simulink model "breathing_rate_adc1"  (R2020b)
settings: Solver=ode15s  StartTime=0.0  StopTime=60  RelTol=1e-3  AbsTol=1e-3  EnableMultiTasking=on
undefined symbols (not defined in the file): sigbuilder_block
libraries: fl_lib x22, nesl_utility x6, ee_lib x4, simulink x1
CloseFcn:
  | try,close(h1_elec_strain_gauge),end
  | clear h1_elec_strain_gauge
  | 
  | clear logsout_elec_strain_gauge
  | clear simlog_elec_strain_gauge
  | clear tout
Description:
  | Strain Gauge and Wheatstone Bridge
  | 
  | Copyright 2008-2018 The MathWorks, Inc.
settings Model: ExtModeAutoUpdateStatusClock=off  Creator=MathWorks  LastModifiedBy=bolic
settings SolverCC: AutoScaleAbsTol=off
settings DataIOCC: MaxDataPoints=10000  ReturnWorkspaceOutputs=off  SignalLoggingName=logsout_elec_strain_gauge  Refine=5
settings OptimizationCC: ExpressionDepthLimit=2147483647  InitFltsAndDblsToZero=on  LifeSpan=inf
settings DebuggingCC: SaveWithParameterizedLinksMsg=none  UnderspecifiedInitializationDetection=Classic  MergeDetectMultiDrivingBlocksExec=none  SignalResolutionControl=TryResolveAllWithWarning  FcnCallInpInsideContextMsg=warning  StateNameClashWarn=warning  SFUnexpectedBacktrackingDiag=warning  SFNoUnconditionalDefaultTransitionDiag=warning  SFExecutionAtInitializationDiag=none  ArithmeticOperatorsInVariantConditions=warning
settings HardwareCC: ProdBitPerPointer=32  ProdBitPerSizeT=32  ProdBitPerPtrDiffT=32  ProdLargestAtomicFloat=None  ProdIntDivRoundTo=Undefined  ProdEndianess=Unspecified  ProdWordSize=32  ProdHWDeviceType=32-bit Generic
settings ModelReferenceCC: PropagateSignalLabelsOutOfModel=off
settings SFSimCC: SimUseLocalCustomCode=off  CustomCodeUndefinedFunction=UseInterfaceOnly
settings RTWCC: RTWUseLocalCustomCode=off
settings CodeAppCC: StateflowObjectComments=on
settings GRTTargetCC: TargetFcnLib=ansi_tfl_tmw.mat  TargetLangStandard=C89/C90 (ANSI)  CombineOutputUpdateFcns=off  GRTInterface=on
settings ConfigComp: CovMetricSettings=dw  CovSaveCumulativeToWorkspaceVar=on  CovSaveSingleToWorkspaceVar=on  CovExternalEMLEnable=off  CovSFcnEnable=off
settings SimscapeCC: SimscapeLogType=all  SimscapeLogSimulationStatistics=on  SimscapeLogName=simlog_elec_strain_gauge  SimscapeLogDataHistory=10000

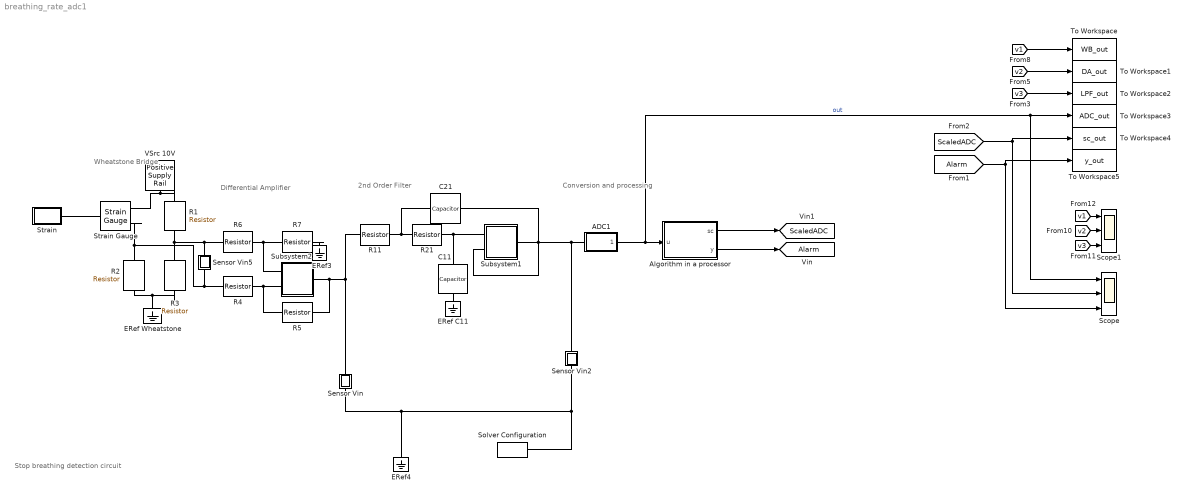
== system breathing_rate_adc1 ==
  note: Differential Amplifier
  note: Wheatstone
      | Bridge
  note: Stop breathing detection circuit
  note: 2nd Order Filter
  note: Conversion and processing
  ADC1 : Subsystem  mask(ADC){fs=80, N=12, vmax=5, ileak=1e-9, C=10e-12}
      mask prompts: fs "Sampling rate (Hz)"; N "Number of bits"; vmax "Input voltage for max output (V)"; ileak "Leakage current (A)"; C "Pin capacitance (F)"
      mask help: Simplified analog-to-digital converter
  Algorithm in a processor : MATLAB Function  TreatAsAtomicUnit=on
  C11 : fl_lib/Electrical/Electrical Elements/Capacitor  c=800 nF  r=0 Ohm  g=0 1/Ohm  i_specify=off  i_priority=High  i=0 A  i_nominal_specify=off  i_nominal_unit=A  i_nominal_value=1  v_specify=off  v_priority=High  v=0 V  v_nominal_specify=off  v_nominal_unit=V  v_nominal_value=1  vc_specify=off  vc_priority=High  vc=0 V  vc_nominal_specify=off  vc_nominal_unit=V  vc_nominal_value=1
      settings: SourceProductName=Foundation Library
  C21 : fl_lib/Electrical/Electrical Elements/Capacitor  c=800 nF  r=0 Ohm  g=0 1/Ohm  i_specify=off  i_priority=High  i=0 A  i_nominal_specify=off  i_nominal_unit=A  i_nominal_value=1  v_specify=off  v_priority=High  v=0 V  v_nominal_specify=off  v_nominal_unit=V  v_nominal_value=1  vc_specify=off  vc_priority=High  vc=0 V  vc_nominal_specify=off  vc_nominal_unit=V  vc_nominal_value=1
      settings: SourceProductName=Foundation Library
  ERef C11 : fl_lib/Electrical/Electrical Elements/Electrical Reference
      settings: SourceProductName=Foundation Library
  ERef Wheatstone : fl_lib/Electrical/Electrical Elements/Electrical Reference
      settings: SourceProductName=Foundation Library
  ERef3 : fl_lib/Electrical/Electrical Elements/Electrical Reference
      settings: SourceProductName=Foundation Library
  ERef4 : fl_lib/Electrical/Electrical Elements/Electrical Reference
      settings: SourceProductName=Foundation Library
  R{1..4,6} (5 alike) : fl_lib/Electrical/Electrical Elements/Resistor  R=100 Ohm  i_specify=off  i_priority=High  i=0 A  i_nominal_specify=off  i_nominal_unit=A  i_nominal_value=1  v_specify=off  v_priority=High  v=0 V  v_nominal_specify=off  v_nominal_unit=V  v_nominal_value=1
      settings: SourceProductName=Foundation Library
  R11 : fl_lib/Electrical/Electrical Elements/Resistor  R=10 kOhm  i_specify=off  i_priority=High  i=0 A  i_nominal_specify=off  i_nominal_unit=A  i_nominal_value=1  v_specify=off  v_priority=High  v=0 V  v_nominal_specify=off  v_nominal_unit=V  v_nominal_value=1
      settings: SourceProductName=Foundation Library
  R21 : fl_lib/Electrical/Electrical Elements/Resistor  R="10  kOhm"  i_specify=off  i_priority=High  i=0 A  i_nominal_specify=off  i_nominal_unit=A  i_nominal_value=1  v_specify=off  v_priority=High  v=0 V  v_nominal_specify=off  v_nominal_unit=V  v_nominal_value=1
      settings: SourceProductName=Foundation Library
  R5 : fl_lib/Electrical/Electrical Elements/Resistor  R=10 kOhm  i_specify=off  i_priority=High  i=0 A  i_nominal_specify=off  i_nominal_unit=A  i_nominal_value=1  v_specify=off  v_priority=High  v=0 V  v_nominal_specify=off  v_nominal_unit=V  v_nominal_value=1
      settings: SourceProductName=Foundation Library
  R7 : fl_lib/Electrical/Electrical Elements/Resistor  R=10 kOhm  i_specify=off  i_priority=High  i=0 A  i_nominal_specify=off  i_nominal_unit=A  i_nominal_value=1  v_specify=off  v_priority=High  v=0 V  v_nominal_specify=off  v_nominal_unit=V  v_nominal_value=1
      settings: SourceProductName=Foundation Library
  Scope : Scope  NumInputPorts=3
  Scope1 : Scope  NumInputPorts=3
  Sensor Vin : Subsystem
      mask Display: disp('v')
  Sensor Vin2 : Subsystem
      mask Display: disp('v')
  Sensor Vin5 : Subsystem
      mask Display: disp('v')
  Solver Configuration : nesl_utility/Solver Configuration  PhysicalDomain=network_engine_domain  SubClassName=solver  LeftPortType=input  RightPortType=generic  Tones=[]  Harmonics=[]  SimulateNoise=off  Profile=off  UseLocalSampling=off  EnableSwitchedLinearOptims=on  FrequencyDomain=off  UseCCode=off  RelTol=0.001  AbsTol=1e-06  MinStep=1e-09  ToWorkspace=off  RevertToSquareIcSolve=off  NumHomotopyIterations=100  PhasorMode=off  PhasorModeNumHarmonics=1  DoDC=off  ResidualTolerance=1e-9  UseLocalSolver=off  LocalSolverChoice=NE_BACKWARD_EULER_ADVANCER  LocalSolverSampleTime=.001  DoFixedCost=off  MaxNonlinIter=3  MaxModeIter=2  ComputeImpulses=off  ImpulseIterations=2  LinearAlgebra=auto  EquationFormulation=NE_TIME_EF  DelaysMemoryBudget=1024  AutomaticFiltering=on  FilteringTimeConstant=0.001  PartitionStorageMethod=AS_NEEDED  PartitionMemoryBudget=1024  PartitionMethod=FAST
  Strain : Subsystem
      mask Display: disp('Input')
  Strain Gauge : ee_lib/Sensors & Transducers/Strain Gauge  R=100 Ohm  K=2
      settings: SourceProductBaseCode=PS  InternalSimscapePortConfiguration="{\"Bottom\":[],\"Left\":[{\"id\":\"E\",\"label\":\"E\",\"type\":\"input\"}],\"Right\":[{\"id\":\"p\",\"label\":\"+\",\"type\":\"foundation.electrical.electrical\"},{\"id\":\"n\",\"label\":\"-\",\"type\":\"foundation.electrical.electrical\"}],\"Top\":[]}"
  Subsystem1 : Subsystem
      mask Display: image('op_amp_plus_up.png')
  Subsystem2 : Subsystem
      mask Display: image('op_amp_plus_up.png')
  To Workspace : ToWorkspace  VariableName=WB_out  SaveFormat=Timeseries  SampleTime=-1
  To Workspace1 : ToWorkspace  VariableName=DA_out  SaveFormat=Timeseries  SampleTime=-1
  To Workspace2 : ToWorkspace  VariableName=LPF_out  SaveFormat=Timeseries  SampleTime=-1
  To Workspace3 : ToWorkspace  VariableName=ADC_out  SaveFormat=Timeseries  SampleTime=-1
  To Workspace4 : ToWorkspace  VariableName=sc_out  SaveFormat=Timeseries  SampleTime=-1
  To Workspace5 : ToWorkspace  VariableName=y_out  SaveFormat=Timeseries  SampleTime=-1
  VSrc 10V : ee_lib/Sources/Positive Supply Rail  v0=5 V
      settings: SourceProductBaseCode=PS  InternalSimscapePortConfiguration="{\"Bottom\":[],\"Left\":[],\"Right\":[{\"id\":\"p\",\"label\":\"\",\"type\":\"foundation.electrical.electrical\"}],\"Top\":[]}"
  tag scope: Alarm=global, ScaledADC=global
  wires:
  [v1] -> To Workspace/1
  [v2] -> To Workspace1/1
  [v3] -> To Workspace2/1
  [v2] -> Scope1/2
  [v3] -> Scope1/3
  [v1] -> Scope1/1
  ADC1/1(Out_Int) -> Scope/1, To Workspace3/1, Algorithm in a processor/1(u)  "out"
  Algorithm in a processor/2(y) -> [Alarm]
  Algorithm in a processor/1(sc) -> [ScaledADC]
  [Alarm] -> To Workspace5/1, Scope/3
  [ScaledADC] -> To Workspace4/1, Scope/2
  connections:
  R1/LConn1 -- Strain Gauge/RConn1 -- VSrc 10V/RConn1
  Strain Gauge/RConn2 -- Sensor Vin5/LConn1 -- R4/LConn1 -- R2/LConn1
  R1/RConn1 -- R6/LConn1 -- Sensor Vin5/RConn1 -- R3/LConn1
  R3/RConn1 -- R2/RConn1 -- ERef Wheatstone/LConn1
  R4/RConn1 -- Subsystem2/LConn2 -- R5/LConn1
  R5/RConn1 -- R11/LConn1 -- Sensor Vin/RConn1 -- Subsystem2/RConn1
  R6/RConn1 -- Subsystem2/LConn1 -- R7/LConn1
  R7/RConn1 -- ERef3/LConn1
  ERef4/LConn1 -- Solver Configuration/RConn1 -- Sensor Vin2/LConn1 -- Sensor Vin/LConn1
  C11/LConn1 -- Subsystem1/LConn1 -- R21/RConn1
  Sensor Vin2/RConn1 -- ADC1/LConn1 -- Subsystem1/LConn2 -- C21/RConn1 -- Subsystem1/RConn1
  C21/LConn1 -- R21/LConn1 -- R11/RConn1
  ERef C11/LConn1 -- C11/RConn1
  Strain/RConn1 -- Strain Gauge/LConn1

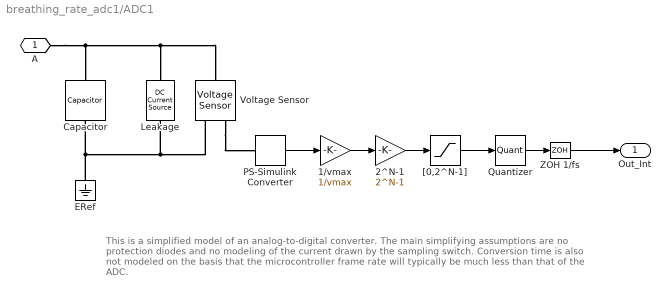
== system breathing_rate_adc1/ADC1 ==
  note: This is a simplified model of an analog-to-digital converter. The main simplifying assumptions
      | are no protection diodes and no modeling of the current drawn by the sampling switch.
      | Conversion time is also not modeled on the basis that the microcontroller frame rate will
      | typically be much less than that of the ADC.
  1/vmax : Gain  Gain=1/vmax
  2^N-1 : Gain  Gain=2^N-1
  Capacitor : fl_lib/Electrical/Electrical Elements/Capacitor  c=1e-6 F  r=1e-6 Ohm  g=0 1/Ohm  i_specify=off  i_priority=High  i=0 A  i_nominal_specify=off  i_nominal_unit=A  i_nominal_value=1  v_specify=off  v_priority=High  v=0 V  v_nominal_specify=off  v_nominal_unit=V  v_nominal_value=1  vc_specify=on  vc_priority=High  vc=0 V  vc_nominal_specify=off  vc_nominal_unit=V  vc_nominal_value=1
      settings: SourceProductName=Foundation Library
  ERef : fl_lib/Electrical/Electrical Elements/Electrical Reference
      settings: SourceProductName=Foundation Library
  Leakage : fl_lib/Electrical/Electrical Sources/DC Current Source  i0=ileak A
      settings: SourceProductName=Foundation Library  InternalSimscapePortConfiguration="{\"Bottom\":[],\"Left\":[{\"id\":\"p\",\"label\":\"\",\"type\":\"foundation.electrical.electrical\"}],\"Right\":[{\"id\":\"n\",\"label\":\"\",\"type\":\"foundation.electrical.electrical\"}],\"Top\":[]}"
  PS-Simulink Converter : nesl_utility/PS-Simulink Converter  PhysicalDomain=network_engine_domain  SubClassName=ps_output  LeftPortType=input  RightPortType=output  PseudoPeriodic=off  Frequencies=[]  Unit=V  AffineConversion=off
  Quantizer : Quantizer  QuantizationInterval=1
  Voltage Sensor : fl_lib/Electrical/Electrical Sensors/Voltage Sensor
      settings: SourceProductName=Foundation Library
  ZOH 1/fs : ZeroOrderHold  SampleTime=1/fs
  "[0,2^N-1]" : Saturate  UpperLimit=2^N-1  LowerLimit=0
  A : PMIOPort  Side=Left
  Out_Int : Outport  VectorParamsAs1DForOutWhenUnconnected=off
  wires:
  "[0,2^N-1]"/1 -> Quantizer/1
  1/vmax/1 -> 2^N-1/1
  2^N-1/1 -> "[0,2^N-1]"/1
  PS-Simulink Converter/1 -> 1/vmax/1
  ZOH 1/fs/1 -> Out_Int/1
  Quantizer/1 -> ZOH 1/fs/1
  connections:
  A/RConn1 -- Voltage Sensor/LConn1 -- Leakage/RConn1 -- Capacitor/LConn1
  ERef/LConn1 -- Voltage Sensor/RConn2 -- Leakage/LConn1 -- Capacitor/RConn1
  Voltage Sensor/RConn1 -- PS-Simulink Converter/LConn1

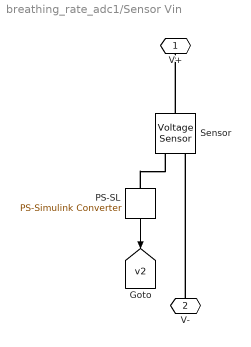
== system breathing_rate_adc1/Sensor Vin ==
  PS-SL : nesl_utility/PS-Simulink Converter  PhysicalDomain=network_engine_domain  SubClassName=ps_output  LeftPortType=input  RightPortType=output  PseudoPeriodic=off  Frequencies=[]  Unit=1  AffineConversion=off
  Sensor : fl_lib/Electrical/Electrical Sensors/Voltage Sensor
      settings: SourceProductName=Foundation Library
  V+ : PMIOPort  Side=Right
  V- : PMIOPort  Port=2  Side=Left
  tag scope: v2=global
  wires:
  PS-SL/1 -> [v2]
  connections:
  PS-SL/LConn1 -- Sensor/RConn1
  Sensor/LConn1 -- V+/RConn1
  V-/RConn1 -- Sensor/RConn2

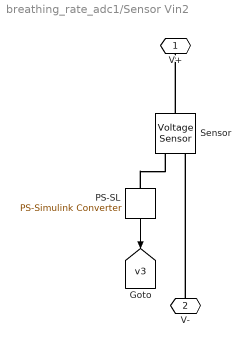
== system breathing_rate_adc1/Sensor Vin2 ==
  PS-SL : nesl_utility/PS-Simulink Converter  PhysicalDomain=network_engine_domain  SubClassName=ps_output  LeftPortType=input  RightPortType=output  PseudoPeriodic=off  Frequencies=[]  Unit=1  AffineConversion=off
  Sensor : fl_lib/Electrical/Electrical Sensors/Voltage Sensor
      settings: SourceProductName=Foundation Library
  V+ : PMIOPort  Side=Right
  V- : PMIOPort  Port=2  Side=Left
  tag scope: v3=global
  wires:
  PS-SL/1 -> [v3]
  connections:
  PS-SL/LConn1 -- Sensor/RConn1
  Sensor/LConn1 -- V+/RConn1
  V-/RConn1 -- Sensor/RConn2

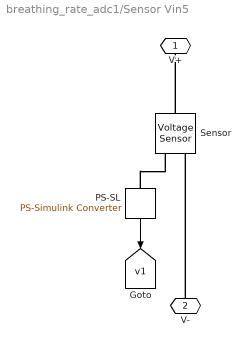
== system breathing_rate_adc1/Sensor Vin5 ==
  PS-SL : nesl_utility/PS-Simulink Converter  PhysicalDomain=network_engine_domain  SubClassName=ps_output  LeftPortType=input  RightPortType=output  PseudoPeriodic=off  Frequencies=[]  Unit=1  AffineConversion=off
  Sensor : fl_lib/Electrical/Electrical Sensors/Voltage Sensor
      settings: SourceProductName=Foundation Library
  V+ : PMIOPort  Side=Right
  V- : PMIOPort  Port=2  Side=Left
  tag scope: v1=global
  wires:
  PS-SL/1 -> [v1]
  connections:
  PS-SL/LConn1 -- Sensor/RConn1
  Sensor/LConn1 -- V+/RConn1
  V-/RConn1 -- Sensor/RConn2

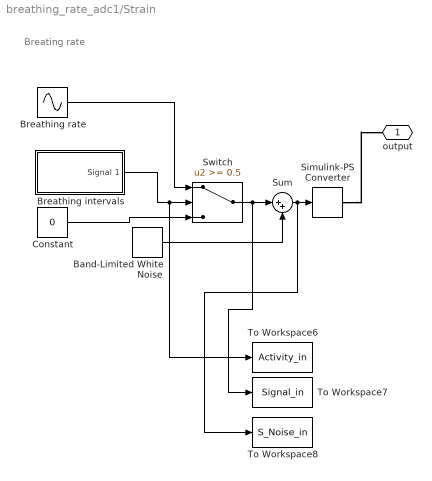
== system breathing_rate_adc1/Strain ==
  note: Breating rate
  Band-Limited White Noise : simulink/Sources/Band-Limited White Noise  Cov=[0.0000000001]  Ts=0.001  seed=[23341]
  Breathing intervals : Subsystem  Tag=STV Subsys  LoadFcn=sigbuilder_block('load');  StartFcn=sigbuilder_block('start');  StopFcn=sigbuilder_block('stop');  ClipboardFcn=sigbuilder_block('clipboard');  mask(Sigbuilder block){tuvar=[0:10]}
      mask help: Simulink:masks:SigbuilderBlock_MD
      mask init:
      | if ~strcmp(get_param(bdroot(gcbh),'SimulationStatus'),'stopped') tuvar = sigbuilder_block('maskInit'); end
      settings: CopyFcn=sigbuilder_block('copy');  DeleteFcn=sigbuilder_block('delete');  ModelCloseFcn=sigbuilder_block('modelClose');  PreSaveFcn=sigbuilder_block('preSave');  PauseFcn=sigbuilder_block('pause');  ContinueFcn=sigbuilder_block('continue');  NameChangeFcn=sigbuilder_block('namechange');  OpenFcn=sigbuilder_block('open',[56.3478 1.56522 1148.87 575.217 ]);  CloseFcn=sigbuilder_block('close');
      mask Display: plot(0, 0, 100, 100,[2, 2, 32, 32, 2], [68, 8, 8, 68, 68],[32, 2], [38, 38], [32, 19, 2],[53, 60, 44], [32, 17, 17, 2],[16, 16, 31, 31]);txt = getActiveGroup(gcbh);text(2, 100, txt,'verticalAlignment', 'top');
  Breathing rate : Sin  Amplitude=-0.01  Bias=0.01  Frequency=pi/2  SampleTime=0.001
  Constant : Constant  Value=0
  Simulink-PS Converter : nesl_utility/Simulink-PS Converter  PhysicalDomain=network_engine_domain  SubClassName=ps_input  LeftPortType=input  RightPortType=output  PseudoPeriodic=off  Frequencies=[]  NoiseDistribution=none  NoiseParameters=[]  Unit=1  AffineConversion=off  FilteringAndDerivatives=zero  SimscapeFilterOrder=1  InputFilterTimeConstant=.001  UdotUserProvided=0
  Sum : Sum  Inputs=|++
  Switch : Switch  Threshold=0.5
  To Workspace6 : ToWorkspace  VariableName=Activity_in  SaveFormat=Timeseries  SampleTime=-1
  To Workspace7 : ToWorkspace  VariableName=Signal_in  SaveFormat=Timeseries  SampleTime=-1
  To Workspace8 : ToWorkspace  VariableName=S_Noise_in  SaveFormat=Timeseries  SampleTime=-1
  output : PMIOPort  Side=Right
  wires:
  Breathing rate/1 -> Switch/1
  Band-Limited White Noise/1 -> Sum/2
  Constant/1 -> Switch/3
  Sum/1 -> To Workspace8/1, Simulink-PS Converter/1
  Switch/1 -> To Workspace7/1, Sum/1
  Breathing intervals/1(Signal 1) -> To Workspace6/1, Switch/2
  connections:
  Simulink-PS Converter/RConn1 -- output/RConn1

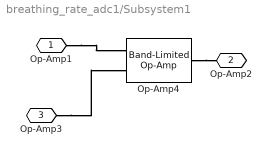
== system breathing_rate_adc1/Subsystem1 ==
  Op-Amp4 : ee_lib/Integrated Circuits/Band-Limited Op-Amp  A=50000  Rin=6e+6 Ohm  Rout=100 Ohm  Vmin=-5 V  Vmax=5 V  Vdotmax=0.7e6 V/s  f=1.5e+6 Hz  V0=0 V
      settings: SourceProductBaseCode=SN
  Op-Amp1 : PMIOPort  Side=Left
  Op-Amp2 : PMIOPort  Port=2  Side=Right
  Op-Amp3 : PMIOPort  Port=3  Side=Left
  connections:
  Op-Amp1/RConn1 -- Op-Amp4/LConn1
  Op-Amp3/RConn1 -- Op-Amp4/LConn2
  Op-Amp4/RConn1 -- Op-Amp2/RConn1

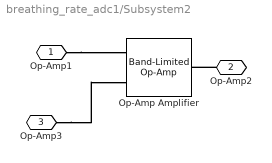
== system breathing_rate_adc1/Subsystem2 ==
  Op-Amp Amplifier : ee_lib/Integrated Circuits/Band-Limited Op-Amp  A=1000000  Rin=1e+06 Ohm  Rout=100 Ohm  Vmin=-5 V  Vmax=5 V  Vdotmax=1000 V/s  f=1e5 Hz  V0=0 V
      settings: SourceProductBaseCode=PS
  Op-Amp1 : PMIOPort  Side=Left
  Op-Amp2 : PMIOPort  Port=2  Side=Right
  Op-Amp3 : PMIOPort  Port=3  Side=Left
  connections:
  Op-Amp1/RConn1 -- Op-Amp Amplifier/LConn1
  Op-Amp3/RConn1 -- Op-Amp Amplifier/LConn2
  Op-Amp2/RConn1 -- Op-Amp Amplifier/RConn1

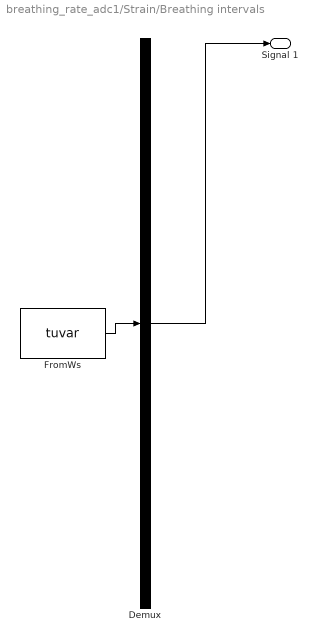
== system breathing_rate_adc1/Strain/Breathing intervals ==
  Demux : Demux  Tag=STV Demux  Outputs=1
      settings: DisplayOption=none
  FromWs : FromWorkspace  Tag=STV FromWs  VariableName=tuvar
      SigBuilderData=|
      | common.afterFinalStr = 'Extrapolate'
      | common.sampleTime = 0
      | dataSet.timeRange = [0 60]
      | dataSet.name = 'Group 1'
      | sbobj.Groups.Name = 'Group 1'
      | sbobj.Groups.Signals.Name = 'Signal 1'
      | sbobj.Groups.Signals.XData = [0 10 10 13 13 24.95 24.95 40 40 48.6 48.6 55 55 60]
      | sbobj.Groups.Signals.YData = [1 1 0 0 1 1 0 0 1 1 0 -0.006 1 1]
      | sbobj.Groups.TimeRange = [0 60]
  Signal 1 : Outport  Tag=STV Outport  VectorParamsAs1DForOutWhenUnconnected=off
  wires:
  Demux/1 -> Signal 1/1
  FromWs/1 -> Demux/1

== matlab function breathing_rate_adc1/Algorithm in a processor ==
  data: sc output; u input; y output
function [sc, y] = alarm(u)
AVERAGING=0;
fs=80;
% Instead of working with buffers, here we store all the scaled data in the
% memory modelled as an array v. Then, when analysing if there is no
% breathing for the time defined by time_for_alarm, we use last
% time_for_alarm samples from the buffer.
% i is also persistent and determines the number of elements that were
% read until this point.
time_for_alarm=10*fs; % 10 sec;
persistent v i
% If persistent variables were not initialized, this means that this is
% the first sample that is being read.
if isempty(i)
    v=zeros(1,100000);
    i=0;
    y=0;
    sc=0;
else
    i=i+1;
    sc = u*5/(2^12-1);  % scale back
    v(i)=sc;            % store the signal into an array v
    if (i>time_for_alarm)
        % simply checking the threshold - sensitive to movement artifatcs
        if AVERAGING ==0
            ind=find(v(i-time_for_alarm+1:i)>0.5);  % if the signal is lower than 0.5 V for more than 10 sec, alarm!
            if isempty(ind)
                y=1;
            else
                y=0;
            end
        else
            % averaging the signal - adding latency
            if mean(v(i-time_for_alarm+1:i))<0.5   % if the mean signal is lower than 0.5 V for more than 10 sec, alarm!
                y=1;
            else
                y=0;
            end
        end
    else
        y=0;
    end
end
